simulink model "ENME403_RotationDynamics"  (R2021a)
settings: Solver=VariableStepAuto  StartTime=0.0  StopTime=10.0  RelTol=1e-3
values from neighbouring files (symbols this model uses):
  C = [eye(3) zeros(3)]    [ENME403_RotationDynamics_sim.m]
  J = diag([1 2 3])    [ENME403_RotationDynamics_sim.m]
settings Model: Creator=Ankit Goel  LastModifiedBy=Ankit Goel

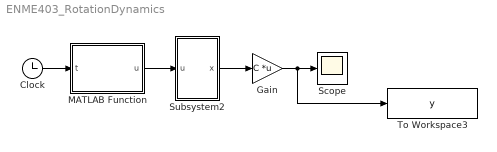
== system ENME403_RotationDynamics ==
  Clock : Clock
  Gain : Gain  Gain=C  Multiplication=Matrix(K*u)
  MATLAB Function : MATLAB Function  TreatAsAtomicUnit=on
  Scope : Scope
  Subsystem2 : Subsystem
  To Workspace3 : ToWorkspace  VariableName=y  SampleTime=-1
  wires:
  Clock/1 -> MATLAB Function/1(t)
  MATLAB Function/1(u) -> Subsystem2/1(u)
  Subsystem2/1(x) -> Gain/1
  Gain/1 -> To Workspace3/1, Scope/1

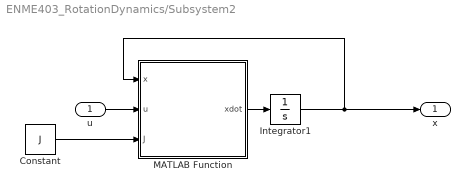
== system ENME403_RotationDynamics/Subsystem2 ==
  u : Inport
  Constant : Constant  Value=J
  Integrator1 : Integrator  InitialCondition=zeros(6,1)
  MATLAB Function : MATLAB Function  TreatAsAtomicUnit=on
  x : Outport
  wires:
  Constant/1 -> MATLAB Function/3(J)
  MATLAB Function/1(xdot) -> Integrator1/1
  Integrator1/1 -> MATLAB Function/1(x), x/1
  u/1 -> MATLAB Function/2(u)

== matlab function ENME403_RotationDynamics/Subsystem2/MATLAB Function ==
  data: x input; u input; xdot output; J input
function xdot = Rotational_dynamics(x,u, J)

Phi     = x(1);
Theta   = x(2);
Psi     = x(3);
omega1  = x(4);
omega2  = x(5);
omega3  = x(6);

xdot        = zeros(6,1);

Phidot      = omega1 + sin(Phi) * tan(Theta) * omega2 + cos(Phi) * tan(Theta) * omega3;
Thetadot    = cos(Phi) * omega2 - sin(Phi) * omega3;
Psidot      = sin(Phi) * sec(Theta) * omega2 + cos(Phi) * sec(Theta) * omega3;

omega       = [omega1; omega2; omega3];
omegadot    = pinv(J)*(-cross(omega, J*omega) + u);

xdot = [Phidot; Thetadot; Psidot; omegadot];
% size(xdot)

== matlab function ENME403_RotationDynamics/MATLAB Function ==
  settings: updateMethod=DISCRETE
  data: t input; u output
function u = input_generator(t)

u = [0.1*sin(3*t);
     0.3*sin(2*t);
     0.2*sin(1*t)];
